simulink model "InterpolationQ"  (R2019b)
settings: Solver=VariableStepDiscrete  StartTime=0.0  StopTime=20  MaxStep=0.01  RelTol=1e-3
undefined symbols (not defined in the file or in its folder): DiscIntNeverNeededParam
settings Model: Creator=Aljaz  LastModifiedBy=Aljaz
settings DataIOCC: SaveOutput=off  SaveTime=off  ReturnWorkspaceOutputs=off

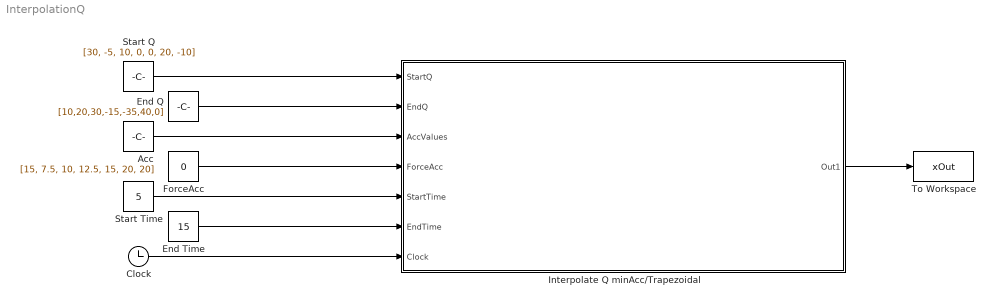
== system InterpolationQ ==
  Acc : Constant  Value=[15, 7.5, 10, 12.5, 15, 20, 20]
  Clock : Clock
  End Q : Constant  Value=[10,20,30,-15,-35,40,0]
  End Time : Constant  Value=15
  ForceAcc : Constant  Value=0
  Interpolate Q minAcc/Trapezoidal : Subsystem
  Start Q : Constant  Value=[30, -5, 10, 0, 0, 20, -10]
  Start Time : Constant  Value=5
  To Workspace : ToWorkspace  VariableName=xOut  SampleTime=-1
  wires:
  Start Q/1 -> Interpolate Q minAcc/Trapezoidal/1(StartQ)
  End Q/1 -> Interpolate Q minAcc/Trapezoidal/2(EndQ)
  Acc/1 -> Interpolate Q minAcc/Trapezoidal/3(AccValues)
  ForceAcc/1 -> Interpolate Q minAcc/Trapezoidal/4(ForceAcc)
  Start Time/1 -> Interpolate Q minAcc/Trapezoidal/5(StartTime)
  End Time/1 -> Interpolate Q minAcc/Trapezoidal/6(EndTime)
  Clock/1 -> Interpolate Q minAcc/Trapezoidal/7(Clock)
  Interpolate Q minAcc/Trapezoidal/1(Out1) -> To Workspace/1

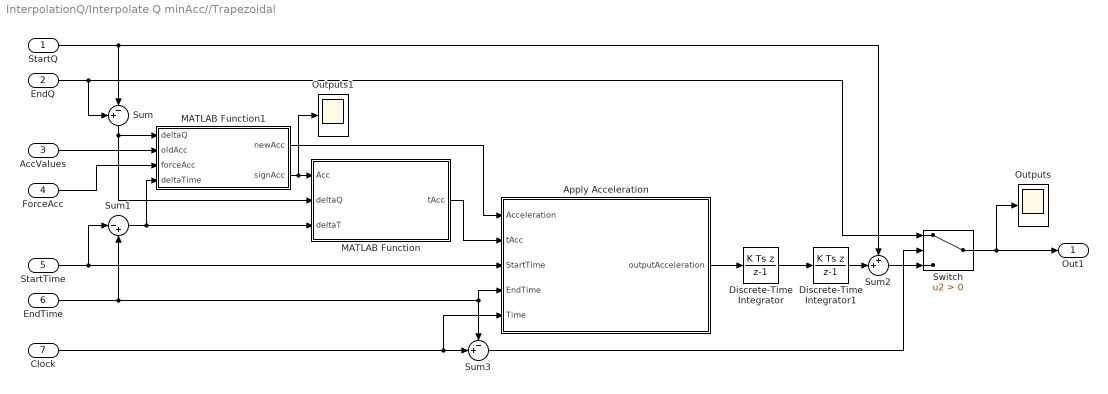
== system InterpolationQ/Interpolate Q minAcc//Trapezoidal ==
  StartQ : Inport
  EndQ : Inport  Port=2
  AccValues : Inport  Port=3
  ForceAcc : Inport  Port=4
  StartTime : Inport  Port=5
  EndTime : Inport  Port=6
  Clock : Inport  Port=7
  Apply Acceleration : Subsystem
  Discrete-Time Integrator : DiscreteIntegrator  IntegratorMethod=Integration: Backward Euler  SampleTime=-1  ICPrevOutput=DiscIntNeverNeededParam  ICPrevScaledInput=DiscIntNeverNeededParam
  Discrete-Time Integrator1 : DiscreteIntegrator  IntegratorMethod=Integration: Backward Euler  SampleTime=-1  ICPrevOutput=DiscIntNeverNeededParam  ICPrevScaledInput=DiscIntNeverNeededParam
  MATLAB Function : MATLAB Function  TreatAsAtomicUnit=on
  MATLAB Function1 : MATLAB Function  TreatAsAtomicUnit=on
  Outputs : Scope
  Outputs1 : Scope
  Sum : Sum  Inputs=+-|
  Sum1 : Sum  Inputs=|-+
  Sum2 : Sum  Inputs=++|
  Sum3 : Sum  Inputs=-+|
  Switch : Switch  Criteria=u2 > Threshold
  Out1 : Outport
  wires:
  EndTime/1 -> Sum3/1, Apply Acceleration/4(EndTime), Sum1/2
  MATLAB Function1/2(signAcc) -> Outputs1/1, MATLAB Function/1(Acc)
  Sum3/1 -> Switch/2
  ForceAcc/1 -> MATLAB Function1/3(forceAcc)
  MATLAB Function/1(tAcc) -> Apply Acceleration/2(tAcc)
  Clock/1 -> Sum3/2, Apply Acceleration/5(Time)
  Sum1/1 -> MATLAB Function1/4(deltaTime), MATLAB Function/3(deltaT)
  Switch/1 -> Out1/1, Outputs/1
  AccValues/1 -> MATLAB Function1/2(oldAcc)
  StartQ/1 -> Sum2/1, Sum/2
  StartTime/1 -> Apply Acceleration/3(StartTime), Sum1/1
  Apply Acceleration/1(outputAcceleration) -> Discrete-Time Integrator/1
  Sum/1 -> MATLAB Function1/1(deltaQ), MATLAB Function/2(deltaQ)
  Discrete-Time Integrator1/1 -> Sum2/2
  Discrete-Time Integrator/1 -> Discrete-Time Integrator1/1
  Sum2/1 -> Switch/3
  EndQ/1 -> Sum/1, Switch/1
  MATLAB Function1/1(newAcc) -> Apply Acceleration/1(Acceleration)

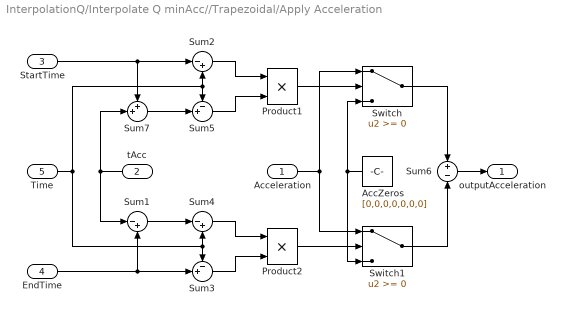
== system InterpolationQ/Interpolate Q minAcc//Trapezoidal/Apply Acceleration ==
  Acceleration : Inport
  tAcc : Inport  Port=2
  StartTime : Inport  Port=3
  EndTime : Inport  Port=4
  Time : Inport  Port=5
  AccZeros : Constant  Value=[0,0,0,0,0,0,0]
  Product1 : Product
  Product2 : Product
  Sum1 : Sum  Inputs=|-+
  Sum2 : Sum  Inputs=|-+
  Sum3 : Sum  Inputs=-+|
  Sum4 : Sum  Inputs=|-+
  Sum5 : Sum  Inputs=-+|
  Sum6 : Sum  Inputs=+|-
  Sum7 : Sum  Inputs=++|
  Switch : Switch
  Switch1 : Switch
  outputAcceleration : Outport
  wires:
  Switch/1 -> Sum6/1
  Acceleration/1 -> Switch/1, Switch1/1
  Switch1/1 -> Sum6/2
  Product1/1 -> Switch/2
  AccZeros/1 -> Switch/3, Switch1/3
  Sum6/1 -> outputAcceleration/1
  Sum2/1 -> Product1/1
  Sum5/1 -> Product1/2
  Time/1 -> Sum4/2, Sum3/1, Sum2/2, Sum5/1
  StartTime/1 -> Sum7/1, Sum2/1
  tAcc/1 -> Sum1/1, Sum7/2
  Sum7/1 -> Sum5/2
  EndTime/1 -> Sum1/2, Sum3/2
  Sum1/1 -> Sum4/1
  Sum4/1 -> Product2/1
  Sum3/1 -> Product2/2
  Product2/1 -> Switch1/2

== matlab function InterpolationQ/Interpolate Q minAcc//Trapezoidal/MATLAB Function1 ==
  data: deltaQ input; oldAcc input; newAcc output; signAcc output; forceAcc input; deltaTime input
function [newAcc,signAcc] = adjustAcc(deltaQ,oldAcc,forceAcc,deltaTime)
if forceAcc~=0
    signAcc=oldAcc.*sign(deltaQ); %adjust sign of acc
else
    tAcc=0.49*deltaTime;
    signAcc=(deltaQ./(deltaTime.*tAcc-tAcc.*tAcc));
end
newAcc=signAcc;%.*0.99012;
end

== matlab function InterpolationQ/Interpolate Q minAcc//Trapezoidal/MATLAB Function ==
  data: Acc input; deltaQ input; tAcc output; deltaT input
function tAcc = getAccTime(Acc,deltaQ,deltaT)

D=deltaT.^2.*Acc-4*deltaQ;
D=D./Acc;
tAcc=deltaT/2-0.5*sqrt(D);
end
